simulink model "Q3_B"  (R2021b)
settings: Solver=VariableStepAuto  StartTime=0.0  StopTime=10  RelTol=1e-3
settings Model: Creator=alimi  LastModifiedBy=alimi

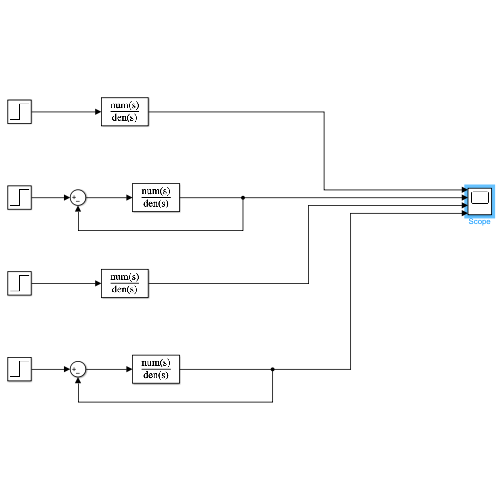
[thumbnail: Simulink's stored preview of the top-level diagram]
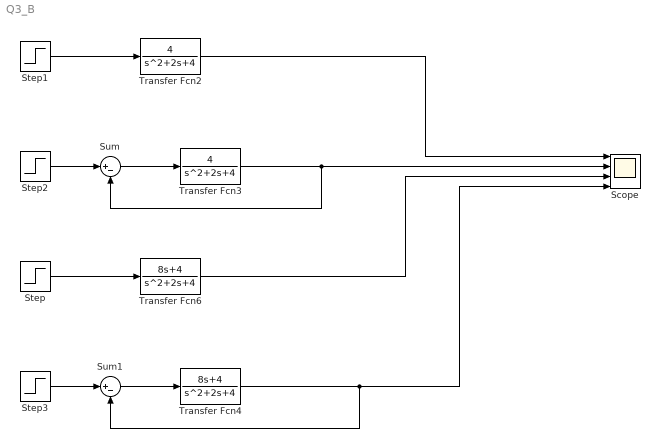
== system Q3_B ==
  Scope : Scope  NumInputPorts=4
  Step{,1..3} (4 alike) : Step  Time=0.001  SampleTime=0
  Sum : Sum  Inputs=|+-
  Sum1 : Sum  Inputs=|+-
  Transfer Fcn2 : TransferFcn  Numerator=[4]  Denominator=[1 2 4]
  Transfer Fcn3 : TransferFcn  Numerator=[4]  Denominator=[1 2 4]
  Transfer Fcn4 : TransferFcn  Numerator=[8 4]  Denominator=[1 2 4]
  Transfer Fcn6 : TransferFcn  Numerator=[8 4]  Denominator=[1 2 4]
  wires:
  Step/1 -> Transfer Fcn6/1
  Step1/1 -> Transfer Fcn2/1
  Transfer Fcn2/1 -> Scope/1
  Step2/1 -> Sum/1
  Sum/1 -> Transfer Fcn3/1
  Transfer Fcn3/1 -> Sum/2, Scope/2
  Sum1/1 -> Transfer Fcn4/1
  Transfer Fcn4/1 -> Scope/4, Sum1/2
  Step3/1 -> Sum1/1
  Transfer Fcn6/1 -> Scope/3
